simulink model "AM-FM"  (R2018a)
settings: Solver=VariableStepAuto  StartTime=0.0  StopTime=0.01  RelTol=1e-3
libraries: dspstat3 x2, dsparch4 x1, simulink x1, dspmathops x1
settings Model: Creator=Asus  LastModifiedBy=Asus

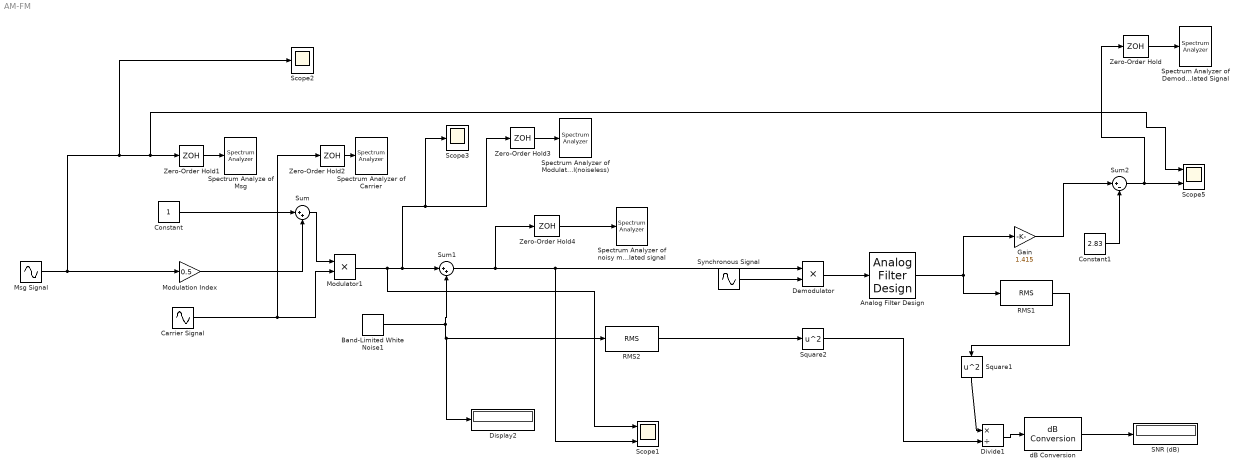
== system AM-FM ==
  Analog Filter Design : dsparch4/Analog Filter Design  method=Butterworth  filttype=Lowpass  N=8  Wlo=2*pi*1000  Whi=80  Rp=2  Rs=40
  Band-Limited White Noise1 : simulink/Sources/Band-Limited White Noise  Cov=[9e-15]  Ts=1/1.35e7  seed=[23341]
  Carrier Signal : Sin  Amplitude=2  Frequency=2*pi*1350000  Phase=pi/2  SampleTime=1/1.35e7
  Constant : Constant
  Constant1 : Constant  Value=2.83
  Demodulator : Product
  Display2 : Display
  Divide1 : Product  Inputs=*/
  Gain : Gain  Gain=1.415
  Modulation Index : Gain  Gain=0.5
  Modulator1 : Product
  Msg Signal : Sin  Frequency=2*pi*1000  Phase=pi/2  SampleTime=1/1.35e7
  RMS1 : dspstat3/RMS  run=off  directionMode=Each column  dimension=1  InputProcessing=Columns as channels (frame based)  reset_popup=None
  RMS2 : dspstat3/RMS  run=off  directionMode=Each column  dimension=1  InputProcessing=Columns as channels (frame based)  reset_popup=None
  SNR (dB) : Display
  Scope1 : Scope  NumInputPorts=2
  Scope2 : Scope
  Scope3 : Scope
  Scope5 : Scope  NumInputPorts=2
  Spectrum Analyze of Msg : SpectrumAnalyzer
  Spectrum Analyzer of Demodulated Signal : SpectrumAnalyzer
  Spectrum Analyzer of Carrier : SpectrumAnalyzer
  Spectrum Analyzer of Modulated Signal(noiseless) : SpectrumAnalyzer
  "Spectrum Analyzer of noisy modulated signal " : SpectrumAnalyzer
  Square1 : Math  Operator=square  SaturateOnIntegerOverflow=on
  Square2 : Math  Operator=square  SaturateOnIntegerOverflow=on
  Sum : Sum  Inputs=|++
  Sum1 : Sum  Inputs=|++
  Sum2 : Sum  Inputs=|+-
  Synchronous Signal : Sin  Amplitude=2  Frequency=2*pi*1350000  Phase=pi/2  SampleTime=1/1.35e7
  Zero-Order Hold{,1..4} (5 alike) : ZeroOrderHold  SampleTime=-1
  dB Conversion : dspmathops/dB Conversion  dBtype=dB  intype=Amplitude  R=1.5e10  fuzz=off
      settings: SourceProductName=DSP System Toolbox
  wires:
  Sum/1 -> Modulator1/1
  Constant/1 -> Sum/1
  Modulation Index/1 -> Sum/2
  Demodulator/1 -> Analog Filter Design/1
  Analog Filter Design/1 -> RMS1/1, Gain/1
  RMS2/1 -> Square2/1
  Square2/1 -> Divide1/2
  Divide1/1 -> dB Conversion/1
  dB Conversion/1 -> SNR (dB)/1
  Synchronous Signal/1 -> Demodulator/2
  Gain/1 -> Sum2/1
  Constant1/1 -> Sum2/2
  Msg Signal/1 -> Scope2/1, Zero-Order Hold1/1, Scope5/1, Modulation Index/1
  Sum2/1 -> Zero-Order Hold/1, Scope5/2
  Zero-Order Hold/1 -> Spectrum Analyzer of Demodulated Signal/1
  Carrier Signal/1 -> Zero-Order Hold2/1, Modulator1/2
  Zero-Order Hold2/1 -> Spectrum Analyzer of Carrier/1
  Modulator1/1 -> Scope1/1, Zero-Order Hold3/1, Scope3/1, Sum1/1
  Sum1/1 -> Zero-Order Hold4/1, Scope1/2, Demodulator/1
  Square1/1 -> Divide1/1
  RMS1/1 -> Square1/1
  Zero-Order Hold3/1 -> Spectrum Analyzer of Modulated Signal(noiseless)/1
  Band-Limited White Noise1/1 -> Sum1/2, Display2/1, RMS2/1
  Zero-Order Hold1/1 -> Spectrum Analyze of Msg/1
  Zero-Order Hold4/1 -> "Spectrum Analyzer of noisy modulated signal "/1
